simulink model "ASDP4"  (R2020b)
settings: Solver=VariableStepAuto  StartTime=0.0  StopTime=10.0  RelTol=1e-3
settings Model: Creator=macra  LastModifiedBy=macra

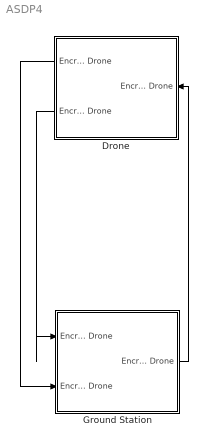
== system ASDP4 ==
  Drone : Subsystem
      settings: PortSchema="{\"entries\":[{\"content\":{\"headerSize\":26,\"margin\":15,\"minimumSpacing\":25,\"sides\":[{\"content\":{\"connectorIds\":[\"Out1\",\"Out2\"]},\"type\":\"ConnectorPlacement.EquallySpacedRectSide\",\"uuid\":\"5dbdb512-c724-4537-b423-e7f241817497\"},{\"content\":{\"connectorIds\":[\"In1\"],\"side\":\"RIGHT\"},\"type\":\"ConnectorPlacement.EquallySpacedRectSide\",\"uuid\":\"ed169a95-4211-4c22-8607-e2cdf6a6fff2\"},{\"content\":{\"connectorIds\":[],\"side\":\"TOP\"},\"type\":\"ConnectorPlacement.EquallySpacedRectSide\",\"uuid\":\"83c28233-b95d-4084-ab80-743a8fa582e0\"},{\"content\":{\"connectorIds\":[],\"side\":\"HIDDEN\"},\"type\":\"ConnectorPlacement.EquallySpacedRectSide\",\"uuid\":\"78dc0539-d843-45d4-8b50-0f9c194c2eeb\"}]},\"type\":\"ConnectorPlacement.EquallySpacedConnector\",\"uuid\":\"65b23c69-016e-4b27-94b8-7f752ac94c38\"}],\"packageUris\":[\"http://schema.mathworks.com/mf0/Connector/R2020b\"],\"version\":\"1.0\"}"
  Ground Station : Subsystem
      settings: PortSchema="{\"entries\":[{\"content\":{\"headerSize\":26,\"margin\":15,\"minimumSpacing\":25,\"sides\":[{\"content\":{\"connectorIds\":[\"In1\",\"In2\"]},\"type\":\"ConnectorPlacement.EquallySpacedRectSide\",\"uuid\":\"5dbdb512-c724-4537-b423-e7f241817497\"},{\"content\":{\"connectorIds\":[\"Out1\"],\"side\":\"RIGHT\"},\"type\":\"ConnectorPlacement.EquallySpacedRectSide\",\"uuid\":\"ed169a95-4211-4c22-8607-e2cdf6a6fff2\"},{\"content\":{\"connectorIds\":[],\"side\":\"TOP\"},\"type\":\"ConnectorPlacement.EquallySpacedRectSide\",\"uuid\":\"83c28233-b95d-4084-ab80-743a8fa582e0\"},{\"content\":{\"connectorIds\":[],\"side\":\"HIDDEN\"},\"type\":\"ConnectorPlacement.EquallySpacedRectSide\",\"uuid\":\"78dc0539-d843-45d4-8b50-0f9c194c2eeb\"}]},\"type\":\"ConnectorPlacement.EquallySpacedConnector\",\"uuid\":\"65b23c69-016e-4b27-94b8-7f752ac94c38\"}],\"packageUris\":[\"http://schema.mathworks.com/mf0/Connector/R2020b\"],\"version\":\"1.0\"}"
  wires:
  Drone/2(Encrypted Data From Drone) -> Ground Station/1(Encrypted Data From Drone)
  Drone/1(Encrypted Video From Drone) -> Ground Station/2(Encrypted Video From Drone)
  Ground Station/1(Encrypted Data To Drone) -> Drone/1(Encrypted Data To Drone)

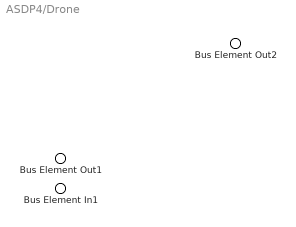
== system ASDP4/Drone ==
  Bus Element In1 : Inport  PortName=Encrypted Data To Drone
  Bus Element Out2 : Outport  PortName=Encrypted Video From Drone
  Bus Element Out1 : Outport  Port=2  PortName=Encrypted Data From Drone

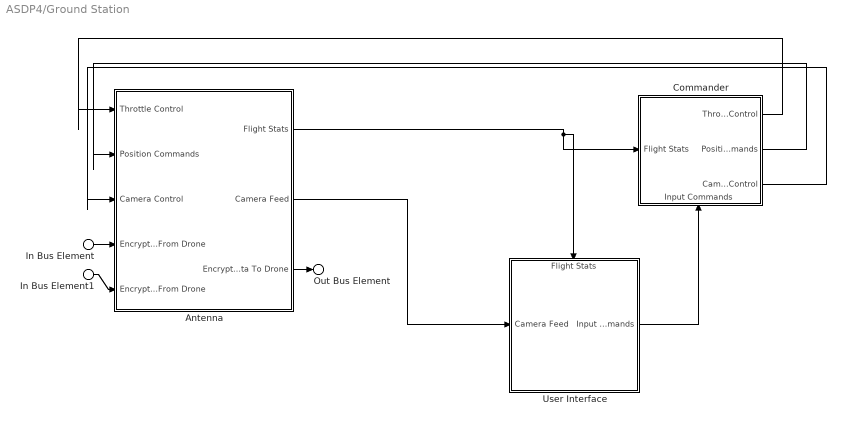
== system ASDP4/Ground Station ==
  In Bus Element : Inport  PortName=Encrypted Data From Drone
  In Bus Element1 : Inport  Port=2  PortName=Encrypted Video From Drone
  Antenna : Subsystem
      settings: PortSchema="{\"entries\":[{\"content\":{\"headerSize\":26,\"margin\":15,\"minimumSpacing\":25,\"sides\":[{\"content\":{\"connectorIds\":[\"In1\",\"In2\",\"In3\",\"In4\",\"In5\"]},\"type\":\"ConnectorPlacement.EquallySpacedRectSide\",\"uuid\":\"8f51257f-f627-4f58-a4af-3e0fb88ba4bc\"},{\"content\":{\"connectorIds\":[\"Out1\",\"Out2\",\"Out3\"],\"side\":\"RIGHT\"},\"type\":\"ConnectorPlacement.EquallySpacedRectSide\",\"uuid\":\"f1fa1950-8e47-40b7-8d13-b3d0804be378\"},{\"content\":{\"connectorIds\":[],\"side\":\"TOP\"},\"type\":\"ConnectorPlacement.EquallySpacedRectSide\",\"uuid\":\"7a27bdc2-dc0c-4d7e-ba2c-0c757f448581\"},{\"content\":{\"connectorIds\":[],\"side\":\"HIDDEN\"},\"type\":\"ConnectorPlacement.EquallySpacedRectSide\",\"uuid\":\"bf1e85f7-7c79-4931-85e3-188682710bd5\"}]},\"type\":\"ConnectorPlacement.EquallySpacedConnector\",\"uuid\":\"5f8c8835-300e-4f03-b548-6a322d546785\"}],\"packageUris\":[\"http://schema.mathworks.com/mf0/Connector/R2020b\"],\"version\":\"1.0\"}"
  Commander : Subsystem
      settings: PortSchema="{\"entries\":[{\"content\":{\"headerSize\":26,\"margin\":15,\"minimumSpacing\":25,\"sides\":[{\"content\":{\"connectorIds\":[\"In1\"]},\"type\":\"ConnectorPlacement.EquallySpacedRectSide\",\"uuid\":\"8f51257f-f627-4f58-a4af-3e0fb88ba4bc\"},{\"content\":{\"connectorIds\":[\"Out1\",\"Out2\",\"Out3\"],\"side\":\"RIGHT\"},\"type\":\"ConnectorPlacement.EquallySpacedRectSide\",\"uuid\":\"f1fa1950-8e47-40b7-8d13-b3d0804be378\"},{\"content\":{\"connectorIds\":[],\"side\":\"TOP\"},\"type\":\"ConnectorPlacement.EquallySpacedRectSide\",\"uuid\":\"7a27bdc2-dc0c-4d7e-ba2c-0c757f448581\"},{\"content\":{\"connectorIds\":[\"In2\"],\"side\":\"BOTTOM\"},\"type\":\"ConnectorPlacement.EquallySpacedRectSide\",\"uuid\":\"100c20a7-19a0-4abc-9a19-4a6d998db79c\"},{\"content\":{\"connectorIds\":[],\"side\":\"HIDDEN\"},\"type\":\"ConnectorPlacement.EquallySpacedRectSide\",\"uuid\":\"bf1e85f7-7c79-4931-85e3-188682710bd5\"}]},\"type\":\"ConnectorPlacement.EquallySpacedConnector\",\"uuid\":\"5f8c8835-300e-4f03-b548-6a322d546785\"}],\"packageUris\":[\"http://schema.mathworks.com/mf0/Connector/R2020b\"],\"version\":\"1.0\"}"
  User Interface : Subsystem
      settings: PortSchema="{\"entries\":[{\"content\":{\"headerSize\":26,\"margin\":15,\"minimumSpacing\":25,\"sides\":[{\"content\":{\"connectorIds\":[\"In2\"]},\"type\":\"ConnectorPlacement.EquallySpacedRectSide\",\"uuid\":\"8f51257f-f627-4f58-a4af-3e0fb88ba4bc\"},{\"content\":{\"connectorIds\":[\"Out1\"],\"side\":\"RIGHT\"},\"type\":\"ConnectorPlacement.EquallySpacedRectSide\",\"uuid\":\"f1fa1950-8e47-40b7-8d13-b3d0804be378\"},{\"content\":{\"connectorIds\":[\"In1\"],\"side\":\"TOP\"},\"type\":\"ConnectorPlacement.EquallySpacedRectSide\",\"uuid\":\"7a27bdc2-dc0c-4d7e-ba2c-0c757f448581\"},{\"content\":{\"connectorIds\":[],\"side\":\"HIDDEN\"},\"type\":\"ConnectorPlacement.EquallySpacedRectSide\",\"uuid\":\"bf1e85f7-7c79-4931-85e3-188682710bd5\"}]},\"type\":\"ConnectorPlacement.EquallySpacedConnector\",\"uuid\":\"5f8c8835-300e-4f03-b548-6a322d546785\"}],\"packageUris\":[\"http://schema.mathworks.com/mf0/Connector/R2020b\"],\"version\":\"1.0\"}"
  Out Bus Element : Outport  PortName=Encrypted Data To Drone
  wires:
  Commander/2(Position Commands) -> Antenna/2(Position Commands)
  Antenna/1(Flight Stats) -> Commander/1(Flight Stats), User Interface/1(Flight Stats)
  Antenna/2(Camera Feed) -> User Interface/2(Camera Feed)
  In Bus Element/1 -> Antenna/4(Encrypted Data From Drone)
  Commander/3(Camera Control) -> Antenna/3(Camera Control)
  User Interface/1(Input Commands) -> Commander/2(Input Commands)
  Antenna/3(Encrypted Data To Drone) -> Out Bus Element/1
  Commander/1(Throttle Control) -> Antenna/1(Throttle Control)
  In Bus Element1/1 -> Antenna/5(Encrypted Video From Drone)

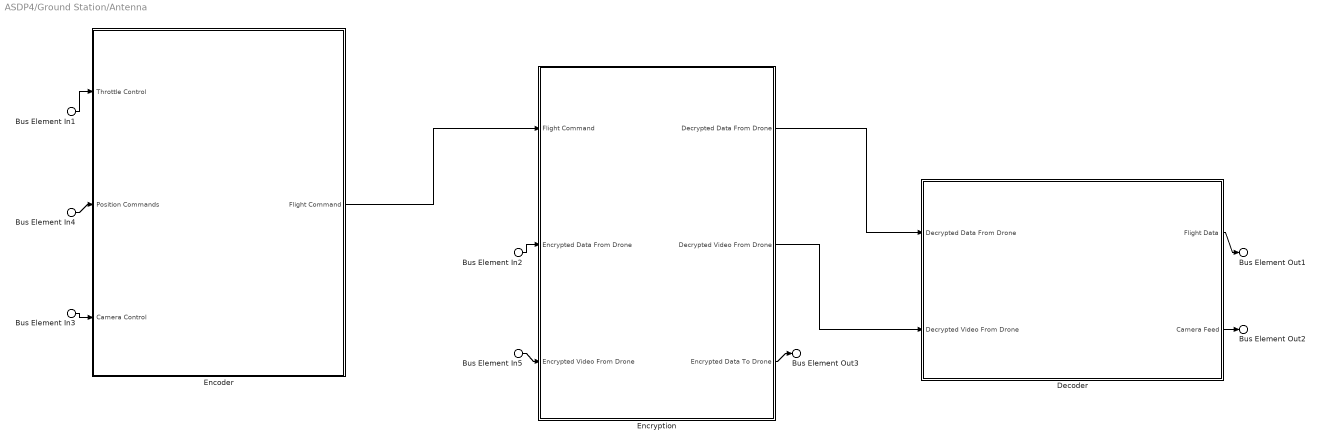
== system ASDP4/Ground Station/Antenna ==
  Bus Element In1 : Inport  PortName=Throttle Control
  Bus Element In4 : Inport  Port=2  PortName=Position Commands
  Bus Element In3 : Inport  Port=3  PortName=Camera Control
  Bus Element In2 : Inport  Port=4  PortName=Encrypted Data From Drone
  Bus Element In5 : Inport  Port=5  PortName=Encrypted Video From Drone
  Decoder : Subsystem
      settings: PortSchema="{\"entries\":[{\"content\":{\"headerSize\":26,\"margin\":15,\"minimumSpacing\":25,\"sides\":[{\"content\":{\"connectorIds\":[\"In1\",\"In2\"]},\"type\":\"ConnectorPlacement.EquallySpacedRectSide\",\"uuid\":\"8f51257f-f627-4f58-a4af-3e0fb88ba4bc\"},{\"content\":{\"connectorIds\":[\"Out1\",\"Out2\"],\"side\":\"RIGHT\"},\"type\":\"ConnectorPlacement.EquallySpacedRectSide\",\"uuid\":\"f1fa1950-8e47-40b7-8d13-b3d0804be378\"},{\"content\":{\"connectorIds\":[],\"side\":\"TOP\"},\"type\":\"ConnectorPlacement.EquallySpacedRectSide\",\"uuid\":\"7a27bdc2-dc0c-4d7e-ba2c-0c757f448581\"},{\"content\":{\"connectorIds\":[],\"side\":\"HIDDEN\"},\"type\":\"ConnectorPlacement.EquallySpacedRectSide\",\"uuid\":\"bf1e85f7-7c79-4931-85e3-188682710bd5\"}]},\"type\":\"ConnectorPlacement.EquallySpacedConnector\",\"uuid\":\"5f8c8835-300e-4f03-b548-6a322d546785\"}],\"packageUris\":[\"http://schema.mathworks.com/mf0/Connector/R2020b\"],\"version\":\"1.0\"}"
  Encoder : Subsystem
      settings: PortSchema="{\"entries\":[{\"content\":{\"headerSize\":26,\"margin\":15,\"minimumSpacing\":25,\"sides\":[{\"content\":{\"connectorIds\":[\"In1\",\"In2\",\"In3\"]},\"type\":\"ConnectorPlacement.EquallySpacedRectSide\",\"uuid\":\"8f51257f-f627-4f58-a4af-3e0fb88ba4bc\"},{\"content\":{\"connectorIds\":[\"Out1\"],\"side\":\"RIGHT\"},\"type\":\"ConnectorPlacement.EquallySpacedRectSide\",\"uuid\":\"f1fa1950-8e47-40b7-8d13-b3d0804be378\"},{\"content\":{\"connectorIds\":[],\"side\":\"TOP\"},\"type\":\"ConnectorPlacement.EquallySpacedRectSide\",\"uuid\":\"7a27bdc2-dc0c-4d7e-ba2c-0c757f448581\"},{\"content\":{\"connectorIds\":[],\"side\":\"HIDDEN\"},\"type\":\"ConnectorPlacement.EquallySpacedRectSide\",\"uuid\":\"bf1e85f7-7c79-4931-85e3-188682710bd5\"}]},\"type\":\"ConnectorPlacement.EquallySpacedConnector\",\"uuid\":\"5f8c8835-300e-4f03-b548-6a322d546785\"}],\"packageUris\":[\"http://schema.mathworks.com/mf0/Connector/R2020b\"],\"version\":\"1.0\"}"
  Encryption : Subsystem
      settings: PortSchema="{\"entries\":[{\"content\":{\"headerSize\":26,\"margin\":15,\"minimumSpacing\":25,\"sides\":[{\"content\":{\"connectorIds\":[\"In1\",\"In2\",\"In3\"]},\"type\":\"ConnectorPlacement.EquallySpacedRectSide\",\"uuid\":\"8f51257f-f627-4f58-a4af-3e0fb88ba4bc\"},{\"content\":{\"connectorIds\":[\"Out1\",\"Out2\",\"Out3\"],\"side\":\"RIGHT\"},\"type\":\"ConnectorPlacement.EquallySpacedRectSide\",\"uuid\":\"f1fa1950-8e47-40b7-8d13-b3d0804be378\"},{\"content\":{\"connectorIds\":[],\"side\":\"TOP\"},\"type\":\"ConnectorPlacement.EquallySpacedRectSide\",\"uuid\":\"7a27bdc2-dc0c-4d7e-ba2c-0c757f448581\"},{\"content\":{\"connectorIds\":[],\"side\":\"HIDDEN\"},\"type\":\"ConnectorPlacement.EquallySpacedRectSide\",\"uuid\":\"bf1e85f7-7c79-4931-85e3-188682710bd5\"}]},\"type\":\"ConnectorPlacement.EquallySpacedConnector\",\"uuid\":\"5f8c8835-300e-4f03-b548-6a322d546785\"}],\"packageUris\":[\"http://schema.mathworks.com/mf0/Connector/R2020b\"],\"version\":\"1.0\"}"
  Bus Element Out1 : Outport  PortName=Flight Stats
  Bus Element Out2 : Outport  Port=2  PortName=Camera Feed
  Bus Element Out3 : Outport  Port=3  PortName=Encrypted Data To Drone
  wires:
  Bus Element In2/1 -> Encryption/2(Encrypted Data From Drone)
  Encryption/3(Encrypted Data To Drone) -> Bus Element Out3/1
  Encryption/1(Decrypted Data From Drone) -> Decoder/1(Decrypted Data From Drone)
  Decoder/1(Flight Data) -> Bus Element Out1/1
  Decoder/2(Camera Feed) -> Bus Element Out2/1
  Encoder/1(Flight Command) -> Encryption/1(Flight Command)
  Bus Element In1/1 -> Encoder/1(Throttle Control)
  Bus Element In3/1 -> Encoder/3(Camera Control)
  Bus Element In5/1 -> Encryption/3(Encrypted Video From Drone)
  Encryption/2(Decrypted Video From Drone) -> Decoder/2(Decrypted Video From Drone)
  Bus Element In4/1 -> Encoder/2(Position Commands)

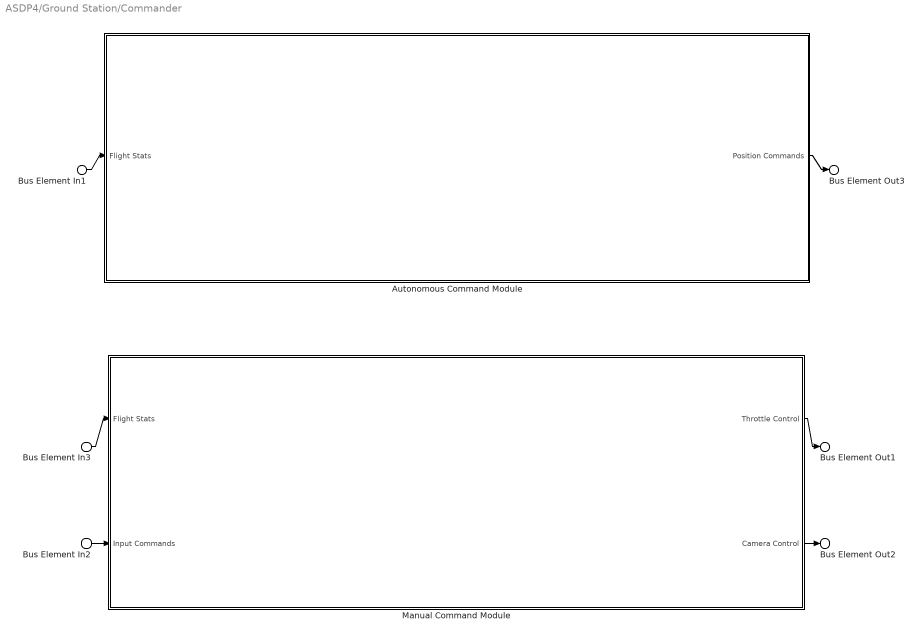
== system ASDP4/Ground Station/Commander ==
  Bus Element In1 : Inport  PortName=Flight Stats
  Bus Element In3 : Inport  PortName=Flight Stats
  Bus Element In2 : Inport  Port=2  PortName=Input Commands
  Autonomous Command Module : Subsystem
      settings: PortSchema="{\"entries\":[{\"content\":{\"headerSize\":26,\"margin\":15,\"minimumSpacing\":25,\"sides\":[{\"content\":{\"connectorIds\":[\"In1\"]},\"type\":\"ConnectorPlacement.EquallySpacedRectSide\",\"uuid\":\"8f51257f-f627-4f58-a4af-3e0fb88ba4bc\"},{\"content\":{\"connectorIds\":[\"Out1\"],\"side\":\"RIGHT\"},\"type\":\"ConnectorPlacement.EquallySpacedRectSide\",\"uuid\":\"f1fa1950-8e47-40b7-8d13-b3d0804be378\"},{\"content\":{\"connectorIds\":[],\"side\":\"TOP\"},\"type\":\"ConnectorPlacement.EquallySpacedRectSide\",\"uuid\":\"7a27bdc2-dc0c-4d7e-ba2c-0c757f448581\"},{\"content\":{\"connectorIds\":[],\"side\":\"HIDDEN\"},\"type\":\"ConnectorPlacement.EquallySpacedRectSide\",\"uuid\":\"bf1e85f7-7c79-4931-85e3-188682710bd5\"}]},\"type\":\"ConnectorPlacement.EquallySpacedConnector\",\"uuid\":\"5f8c8835-300e-4f03-b548-6a322d546785\"}],\"packageUris\":[\"http://schema.mathworks.com/mf0/Connector/R2020b\"],\"version\":\"1.0\"}"
  Manual Command Module : Subsystem
      settings: PortSchema="{\"entries\":[{\"content\":{\"headerSize\":26,\"margin\":15,\"minimumSpacing\":25,\"sides\":[{\"content\":{\"connectorIds\":[\"In1\",\"In2\"]},\"type\":\"ConnectorPlacement.EquallySpacedRectSide\",\"uuid\":\"8f51257f-f627-4f58-a4af-3e0fb88ba4bc\"},{\"content\":{\"connectorIds\":[\"Out1\",\"Out2\"],\"side\":\"RIGHT\"},\"type\":\"ConnectorPlacement.EquallySpacedRectSide\",\"uuid\":\"f1fa1950-8e47-40b7-8d13-b3d0804be378\"},{\"content\":{\"connectorIds\":[],\"side\":\"TOP\"},\"type\":\"ConnectorPlacement.EquallySpacedRectSide\",\"uuid\":\"7a27bdc2-dc0c-4d7e-ba2c-0c757f448581\"},{\"content\":{\"connectorIds\":[],\"side\":\"HIDDEN\"},\"type\":\"ConnectorPlacement.EquallySpacedRectSide\",\"uuid\":\"bf1e85f7-7c79-4931-85e3-188682710bd5\"}]},\"type\":\"ConnectorPlacement.EquallySpacedConnector\",\"uuid\":\"5f8c8835-300e-4f03-b548-6a322d546785\"}],\"packageUris\":[\"http://schema.mathworks.com/mf0/Connector/R2020b\"],\"version\":\"1.0\"}"
  Bus Element Out1 : Outport  PortName=Throttle Control
  Bus Element Out3 : Outport  Port=2  PortName=Position Commands
  Bus Element Out2 : Outport  Port=3  PortName=Camera Control
  wires:
  Bus Element In1/1 -> Autonomous Command Module/1(Flight Stats)
  Bus Element In3/1 -> Manual Command Module/1(Flight Stats)
  Bus Element In2/1 -> Manual Command Module/2(Input Commands)
  Manual Command Module/2(Camera Control) -> Bus Element Out2/1
  Autonomous Command Module/1(Position Commands) -> Bus Element Out3/1
  Manual Command Module/1(Throttle Control) -> Bus Element Out1/1

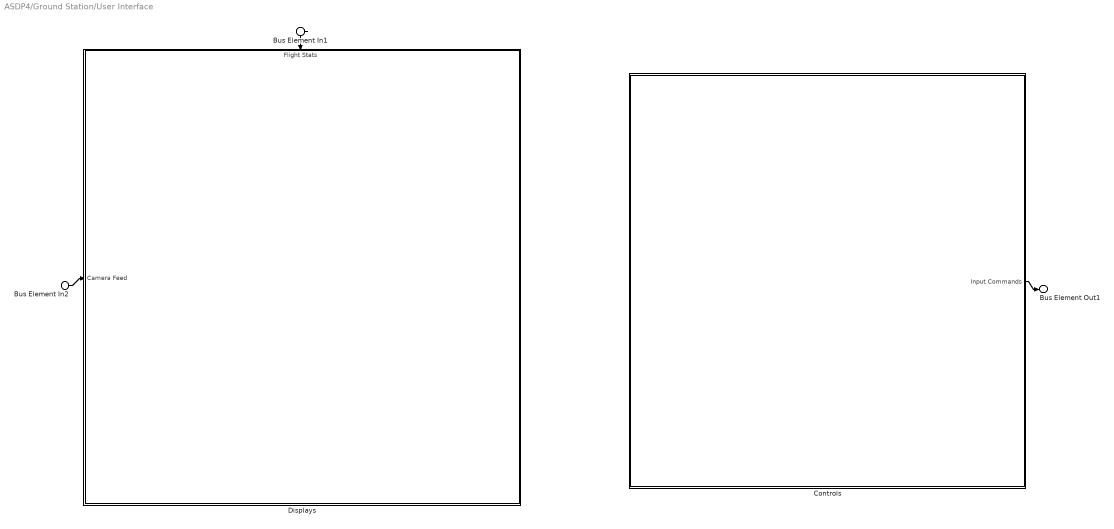
== system ASDP4/Ground Station/User Interface ==
  Bus Element In1 : Inport  PortName=Flight Stats
  Bus Element In2 : Inport  Port=2  PortName=Camera Feed
  Controls : Subsystem
      settings: PortSchema="{\"entries\":[{\"content\":{\"headerSize\":26,\"margin\":15,\"minimumSpacing\":25,\"sides\":[{\"content\":{\"connectorIds\":[]},\"type\":\"ConnectorPlacement.EquallySpacedRectSide\",\"uuid\":\"8f51257f-f627-4f58-a4af-3e0fb88ba4bc\"},{\"content\":{\"connectorIds\":[\"Out1\"],\"side\":\"RIGHT\"},\"type\":\"ConnectorPlacement.EquallySpacedRectSide\",\"uuid\":\"f1fa1950-8e47-40b7-8d13-b3d0804be378\"},{\"content\":{\"connectorIds\":[],\"side\":\"TOP\"},\"type\":\"ConnectorPlacement.EquallySpacedRectSide\",\"uuid\":\"7a27bdc2-dc0c-4d7e-ba2c-0c757f448581\"},{\"content\":{\"connectorIds\":[],\"side\":\"HIDDEN\"},\"type\":\"ConnectorPlacement.EquallySpacedRectSide\",\"uuid\":\"bf1e85f7-7c79-4931-85e3-188682710bd5\"}]},\"type\":\"ConnectorPlacement.EquallySpacedConnector\",\"uuid\":\"5f8c8835-300e-4f03-b548-6a322d546785\"}],\"packageUris\":[\"http://schema.mathworks.com/mf0/Connector/R2020b\"],\"version\":\"1.0\"}"
  Displays : Subsystem
      settings: PortSchema="{\"entries\":[{\"content\":{\"headerSize\":26,\"margin\":15,\"minimumSpacing\":25,\"sides\":[{\"content\":{\"connectorIds\":[\"In1\"]},\"type\":\"ConnectorPlacement.EquallySpacedRectSide\",\"uuid\":\"8f51257f-f627-4f58-a4af-3e0fb88ba4bc\"},{\"content\":{\"connectorIds\":[],\"side\":\"RIGHT\"},\"type\":\"ConnectorPlacement.EquallySpacedRectSide\",\"uuid\":\"f1fa1950-8e47-40b7-8d13-b3d0804be378\"},{\"content\":{\"connectorIds\":[\"In2\"],\"side\":\"TOP\"},\"type\":\"ConnectorPlacement.EquallySpacedRectSide\",\"uuid\":\"7a27bdc2-dc0c-4d7e-ba2c-0c757f448581\"},{\"content\":{\"connectorIds\":[],\"side\":\"HIDDEN\"},\"type\":\"ConnectorPlacement.EquallySpacedRectSide\",\"uuid\":\"bf1e85f7-7c79-4931-85e3-188682710bd5\"}]},\"type\":\"ConnectorPlacement.EquallySpacedConnector\",\"uuid\":\"5f8c8835-300e-4f03-b548-6a322d546785\"}],\"packageUris\":[\"http://schema.mathworks.com/mf0/Connector/R2020b\"],\"version\":\"1.0\"}"
  Bus Element Out1 : Outport  PortName=Input Commands
  wires:
  Bus Element In1/1 -> Displays/2(Flight Stats)
  Bus Element In2/1 -> Displays/1(Camera Feed)
  Controls/1(Input Commands) -> Bus Element Out1/1

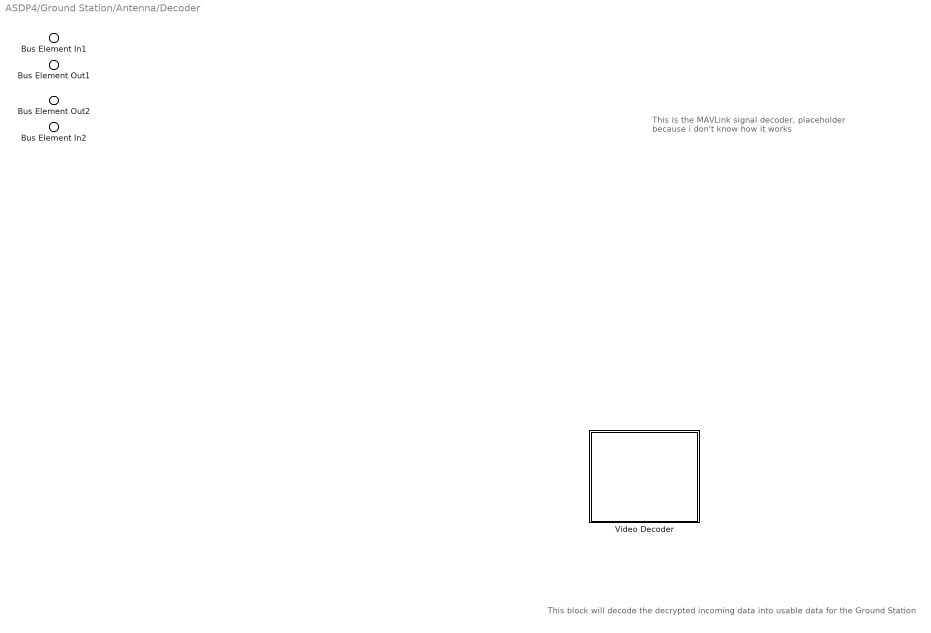
== system ASDP4/Ground Station/Antenna/Decoder ==
  note: This is the MAVLink signal decoder, placeholder
      | because i don't know how it works
  note: This block will decode the decrypted incoming data into usable data for the Ground Station
  Bus Element In1 : Inport  PortName=Decrypted Data From Drone
  Bus Element In2 : Inport  Port=2  PortName=Decrypted Video From Drone
  Video Decoder : Subsystem
      settings: PortSchema="{\"entries\":[{\"content\":{\"headerSize\":26,\"margin\":15,\"minimumSpacing\":25,\"sides\":[{\"content\":{\"connectorIds\":[]},\"type\":\"ConnectorPlacement.EquallySpacedRectSide\",\"uuid\":\"ddae7e39-d932-4e06-be37-e772080feafc\"},{\"content\":{\"connectorIds\":[],\"side\":\"RIGHT\"},\"type\":\"ConnectorPlacement.EquallySpacedRectSide\",\"uuid\":\"8395e97e-bba5-4cd5-932a-1601fa7ff84b\"},{\"content\":{\"connectorIds\":[],\"side\":\"TOP\"},\"type\":\"ConnectorPlacement.EquallySpacedRectSide\",\"uuid\":\"bc67a277-0fbf-4171-9211-28bef4712593\"},{\"content\":{\"connectorIds\":[],\"side\":\"HIDDEN\"},\"type\":\"ConnectorPlacement.EquallySpacedRectSide\",\"uuid\":\"8dbe2d2e-3950-4673-93d1-4d8dcd179cd9\"}]},\"type\":\"ConnectorPlacement.EquallySpacedConnector\",\"uuid\":\"b48a004a-d475-43b1-b758-ab26d47f2dd8\"}],\"packageUris\":[\"http://schema.mathworks.com/mf0/Connector/R2020b\"],\"version\":\"1.0\"}"
  Bus Element Out1 : Outport  PortName=Flight Data
  Bus Element Out2 : Outport  Port=2  PortName=Camera Feed

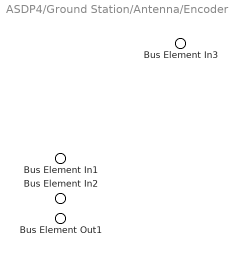
== system ASDP4/Ground Station/Antenna/Encoder ==
  Bus Element In1 : Inport  PortName=Throttle Control
  Bus Element In3 : Inport  Port=2  PortName=Position Commands
  Bus Element In2 : Inport  Port=3  PortName=Camera Control
  Bus Element Out1 : Outport  PortName=Flight Command

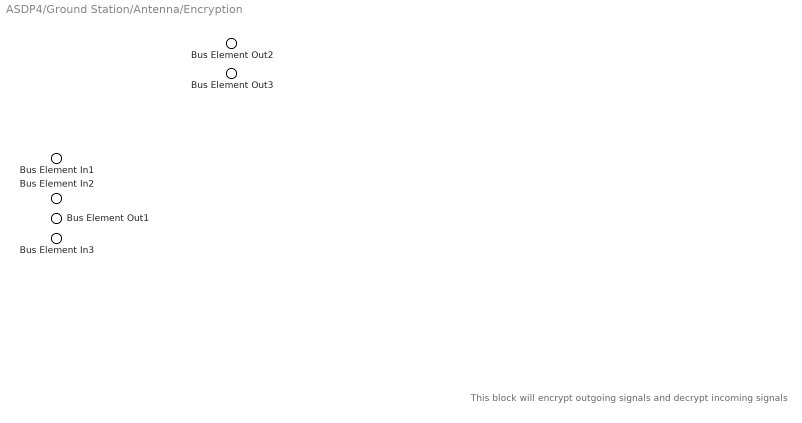
== system ASDP4/Ground Station/Antenna/Encryption ==
  note: This block will encrypt outgoing signals and decrypt incoming signals
  Bus Element In1 : Inport  PortName=Flight Command
  Bus Element In2 : Inport  Port=2  PortName=Encrypted Data From Drone
  Bus Element In3 : Inport  Port=3  PortName=Encrypted Video From Drone
  Bus Element Out2 : Outport  PortName=Decrypted Data From Drone
  Bus Element Out3 : Outport  Port=2  PortName=Decrypted Video From Drone
  Bus Element Out1 : Outport  Port=3  PortName=Encrypted Data To Drone

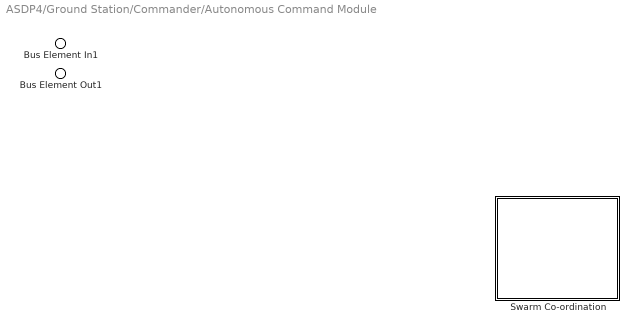
== system ASDP4/Ground Station/Commander/Autonomous Command Module ==
  Bus Element In1 : Inport  PortName=Flight Stats
  Swarm Co-ordination : Subsystem
      settings: PortSchema="{\"entries\":[{\"content\":{\"headerSize\":26,\"margin\":15,\"minimumSpacing\":25,\"sides\":[{\"content\":{\"connectorIds\":[]},\"type\":\"ConnectorPlacement.EquallySpacedRectSide\",\"uuid\":\"ddae7e39-d932-4e06-be37-e772080feafc\"},{\"content\":{\"connectorIds\":[],\"side\":\"RIGHT\"},\"type\":\"ConnectorPlacement.EquallySpacedRectSide\",\"uuid\":\"8395e97e-bba5-4cd5-932a-1601fa7ff84b\"},{\"content\":{\"connectorIds\":[],\"side\":\"TOP\"},\"type\":\"ConnectorPlacement.EquallySpacedRectSide\",\"uuid\":\"bc67a277-0fbf-4171-9211-28bef4712593\"},{\"content\":{\"connectorIds\":[],\"side\":\"HIDDEN\"},\"type\":\"ConnectorPlacement.EquallySpacedRectSide\",\"uuid\":\"8dbe2d2e-3950-4673-93d1-4d8dcd179cd9\"}]},\"type\":\"ConnectorPlacement.EquallySpacedConnector\",\"uuid\":\"b48a004a-d475-43b1-b758-ab26d47f2dd8\"}],\"packageUris\":[\"http://schema.mathworks.com/mf0/Connector/R2020b\"],\"version\":\"1.0\"}"
  Bus Element Out1 : Outport  PortName=Position Commands

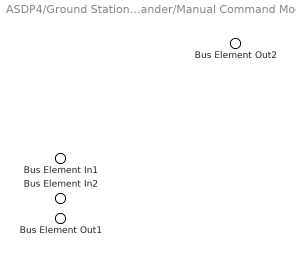
== system ASDP4/Ground Station/Commander/Manual Command Module ==
  Bus Element In1 : Inport  PortName=Flight Stats
  Bus Element In2 : Inport  Port=2  PortName=Input Commands
  Bus Element Out2 : Outport  PortName=Throttle Control
  Bus Element Out1 : Outport  Port=2  PortName=Camera Control

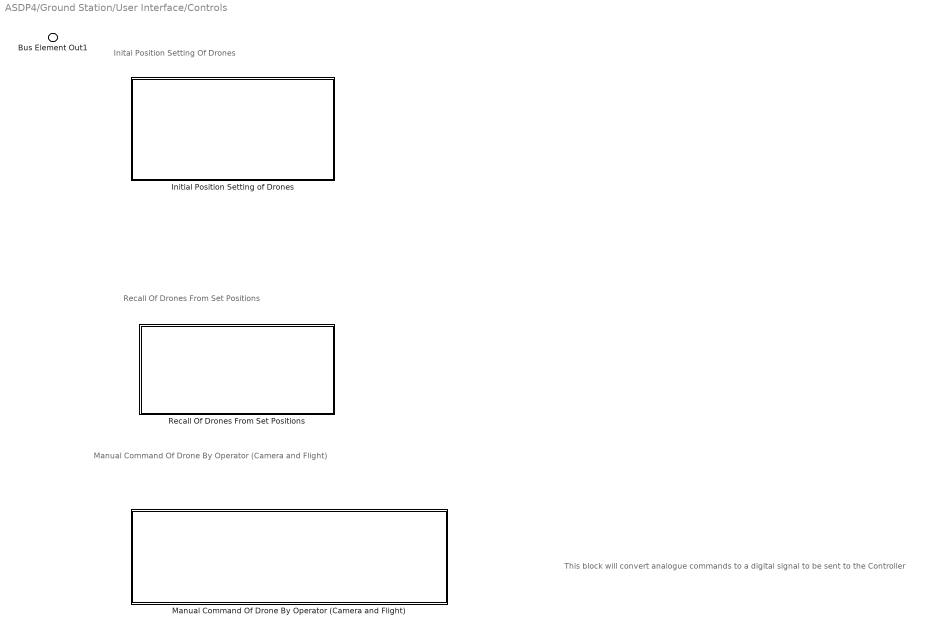
== system ASDP4/Ground Station/User Interface/Controls ==
  note: This block will convert analogue commands to a digital signal to be sent to the Controller
  note: Inital Position Setting Of Drones
  note: Recall Of Drones From Set Positions
  note: Manual Command Of Drone By Operator (Camera and Flight)
  Initial Position Setting of Drones : Subsystem
      settings: PortSchema="{\"entries\":[{\"content\":{\"headerSize\":26,\"margin\":15,\"minimumSpacing\":25,\"sides\":[{\"content\":{\"connectorIds\":[]},\"type\":\"ConnectorPlacement.EquallySpacedRectSide\",\"uuid\":\"ddae7e39-d932-4e06-be37-e772080feafc\"},{\"content\":{\"connectorIds\":[],\"side\":\"RIGHT\"},\"type\":\"ConnectorPlacement.EquallySpacedRectSide\",\"uuid\":\"8395e97e-bba5-4cd5-932a-1601fa7ff84b\"},{\"content\":{\"connectorIds\":[],\"side\":\"TOP\"},\"type\":\"ConnectorPlacement.EquallySpacedRectSide\",\"uuid\":\"bc67a277-0fbf-4171-9211-28bef4712593\"},{\"content\":{\"connectorIds\":[],\"side\":\"HIDDEN\"},\"type\":\"ConnectorPlacement.EquallySpacedRectSide\",\"uuid\":\"8dbe2d2e-3950-4673-93d1-4d8dcd179cd9\"}]},\"type\":\"ConnectorPlacement.EquallySpacedConnector\",\"uuid\":\"b48a004a-d475-43b1-b758-ab26d47f2dd8\"}],\"packageUris\":[\"http://schema.mathworks.com/mf0/Connector/R2020b\"],\"version\":\"1.0\"}"
  Manual Command Of Drone By Operator (Camera and Flight) : Subsystem
      settings: PortSchema="{\"entries\":[{\"content\":{\"headerSize\":26,\"margin\":15,\"minimumSpacing\":25,\"sides\":[{\"content\":{\"connectorIds\":[]},\"type\":\"ConnectorPlacement.EquallySpacedRectSide\",\"uuid\":\"ddae7e39-d932-4e06-be37-e772080feafc\"},{\"content\":{\"connectorIds\":[],\"side\":\"RIGHT\"},\"type\":\"ConnectorPlacement.EquallySpacedRectSide\",\"uuid\":\"8395e97e-bba5-4cd5-932a-1601fa7ff84b\"},{\"content\":{\"connectorIds\":[],\"side\":\"TOP\"},\"type\":\"ConnectorPlacement.EquallySpacedRectSide\",\"uuid\":\"bc67a277-0fbf-4171-9211-28bef4712593\"},{\"content\":{\"connectorIds\":[],\"side\":\"HIDDEN\"},\"type\":\"ConnectorPlacement.EquallySpacedRectSide\",\"uuid\":\"8dbe2d2e-3950-4673-93d1-4d8dcd179cd9\"}]},\"type\":\"ConnectorPlacement.EquallySpacedConnector\",\"uuid\":\"b48a004a-d475-43b1-b758-ab26d47f2dd8\"}],\"packageUris\":[\"http://schema.mathworks.com/mf0/Connector/R2020b\"],\"version\":\"1.0\"}"
  Recall Of Drones From Set Positions : Subsystem
      settings: PortSchema="{\"entries\":[{\"content\":{\"headerSize\":26,\"margin\":15,\"minimumSpacing\":25,\"sides\":[{\"content\":{\"connectorIds\":[]},\"type\":\"ConnectorPlacement.EquallySpacedRectSide\",\"uuid\":\"ddae7e39-d932-4e06-be37-e772080feafc\"},{\"content\":{\"connectorIds\":[],\"side\":\"RIGHT\"},\"type\":\"ConnectorPlacement.EquallySpacedRectSide\",\"uuid\":\"8395e97e-bba5-4cd5-932a-1601fa7ff84b\"},{\"content\":{\"connectorIds\":[],\"side\":\"TOP\"},\"type\":\"ConnectorPlacement.EquallySpacedRectSide\",\"uuid\":\"bc67a277-0fbf-4171-9211-28bef4712593\"},{\"content\":{\"connectorIds\":[],\"side\":\"HIDDEN\"},\"type\":\"ConnectorPlacement.EquallySpacedRectSide\",\"uuid\":\"8dbe2d2e-3950-4673-93d1-4d8dcd179cd9\"}]},\"type\":\"ConnectorPlacement.EquallySpacedConnector\",\"uuid\":\"b48a004a-d475-43b1-b758-ab26d47f2dd8\"}],\"packageUris\":[\"http://schema.mathworks.com/mf0/Connector/R2020b\"],\"version\":\"1.0\"}"
  Bus Element Out1 : Outport  PortName=Input Commands

== system ASDP4/Ground Station/User Interface/Displays ==
  note: This block will display the data from the drone on the operator's monitors
  Bus Element In2 : Inport  PortName=Camera Feed
  Bus Element In1 : Inport  Port=2  PortName=Flight Stats
  Display Customization : Subsystem
      settings: PortSchema="{\"entries\":[{\"content\":{\"headerSize\":26,\"margin\":15,\"minimumSpacing\":25,\"sides\":[{\"content\":{\"connectorIds\":[]},\"type\":\"ConnectorPlacement.EquallySpacedRectSide\",\"uuid\":\"8f51257f-f627-4f58-a4af-3e0fb88ba4bc\"},{\"content\":{\"connectorIds\":[],\"side\":\"RIGHT\"},\"type\":\"ConnectorPlacement.EquallySpacedRectSide\",\"uuid\":\"f1fa1950-8e47-40b7-8d13-b3d0804be378\"},{\"content\":{\"connectorIds\":[],\"side\":\"TOP\"},\"type\":\"ConnectorPlacement.EquallySpacedRectSide\",\"uuid\":\"7a27bdc2-dc0c-4d7e-ba2c-0c757f448581\"},{\"content\":{\"connectorIds\":[],\"side\":\"HIDDEN\"},\"type\":\"ConnectorPlacement.EquallySpacedRectSide\",\"uuid\":\"bf1e85f7-7c79-4931-85e3-188682710bd5\"}]},\"type\":\"ConnectorPlacement.EquallySpacedConnector\",\"uuid\":\"5f8c8835-300e-4f03-b548-6a322d546785\"}],\"packageUris\":[\"http://schema.mathworks.com/mf0/Connector/R2020b\"],\"version\":\"1.0\"}"

== system ASDP4/Ground Station/Antenna/Decoder/Video Decoder ==

== system ASDP4/Ground Station/Commander/Autonomous Command Module/Swarm Co-ordination ==

== system ASDP4/Ground Station/User Interface/Controls/Initial Position Setting of Drones ==

== system ASDP4/Ground Station/User Interface/Controls/Manual Command Of Drone By Operator (Camera and Flight) ==

== system ASDP4/Ground Station/User Interface/Controls/Recall Of Drones From Set Positions ==

== system ASDP4/Ground Station/User Interface/Displays/Display Customization ==
  note: This block will allow the display configuration to be customized
